simulink model "ensembleSNN_simulink"  (R2019a)
settings: Solver=FixedStepAuto  StartTime=0.0  StopTime=12  FixedStep=0.001  RelTol=1e-3
libraries: simulink x2, dspsigops x1
(part 3 of 3)

== system ensembleSNN_simulink/izhiekvichNeuron6/u' switch ==
  In1 : Inport
  In2 : Inport  Port=2
  In3 : Inport  Port=3
  Switch Delay - 3 : Delay  DelayLength=3
  Switch4 : Switch  Criteria=u2 > Threshold  Threshold=30
  Out1 : Outport  VectorParamsAs1DForOutWhenUnconnected=on
  wires:
  In2/1 -> Switch4/2
  Switch4/1 -> Switch Delay - 3/1
  In1/1 -> Switch4/1
  Switch Delay - 3/1 -> Out1/1
  In3/1 -> Switch4/3

== system ensembleSNN_simulink/izhiekvichNeuron6/v + [0.04v2 +5v - u + j +140 ==
  In1 : Inport
  J : Inport  Port=2
  Add : Sum
  Add Delay - 2 : Delay
  Out1 : Outport  VectorParamsAs1DForOutWhenUnconnected=on
  wires:
  Add Delay - 2/1 -> Out1/1
  Add/1 -> Add Delay - 2/1
  In1/1 -> Add/1
  J/1 -> Add/2

== system ensembleSNN_simulink/izhiekvichNeuron6/v' switch ==
  In1 : Inport
  In2 : Inport  Port=2
  In3 : Inport  Port=3
  Switch Delay - 3 : Delay  DelayLength=3
  Switch4 : Switch  Criteria=u2 > Threshold  Threshold=30
  J : Outport  VectorParamsAs1DForOutWhenUnconnected=on
  wires:
  In2/1 -> Switch4/2
  Switch4/1 -> Switch Delay - 3/1
  In1/1 -> Switch4/1
  Switch Delay - 3/1 -> J/1
  In3/1 -> Switch4/3

== system ensembleSNN_simulink/izhiekvichNeuron6/v^2 ==
  J : Inport
  In2 : Inport  Port=2
  Mult Delay - 2 : Delay  DelayLength=1
  Product1 : Product
  Out1 : Outport  VectorParamsAs1DForOutWhenUnconnected=on
  wires:
  Product1/1 -> Mult Delay - 2/1
  In2/1 -> Product1/2
  J/1 -> Product1/1
  Mult Delay - 2/1 -> Out1/1

== system ensembleSNN_simulink/izhiekvichNeuron7/0.04v2 +5v - u ==
  In1 : Inport
  In2 : Inport  Port=2
  Subtract : Sum  Inputs=+-
  Subtract Delay - 1 : Delay  DelayLength=1
  Out1 : Outport  VectorParamsAs1DForOutWhenUnconnected=on
  wires:
  In1/1 -> Subtract/1
  Subtract/1 -> Subtract Delay - 1/1
  Subtract Delay - 1/1 -> Out1/1
  In2/1 -> Subtract/2

== system ensembleSNN_simulink/izhiekvichNeuron7/0.04v2 +5v - u + j +140 ==
  In1 : Inport
  J : Inport  Port=2
  Add : Sum
  Add Delay - 2 : Delay
  Out1 : Outport  VectorParamsAs1DForOutWhenUnconnected=on
  wires:
  Add Delay - 2/1 -> Out1/1
  Add/1 -> Add Delay - 2/1
  In1/1 -> Add/1
  J/1 -> Add/2

== system ensembleSNN_simulink/izhiekvichNeuron7/0.04v^2 ==
  In1 : Inport
  In2 : Inport  Port=2
  Mult Delay - 1 : Delay  DelayLength=1
  Product1 : Product
  Out1 : Outport  VectorParamsAs1DForOutWhenUnconnected=on
  wires:
  Product1/1 -> Mult Delay - 1/1
  Mult Delay - 1/1 -> Out1/1
  In2/1 -> Product1/2
  In1/1 -> Product1/1

== system ensembleSNN_simulink/izhiekvichNeuron7/0.04v^2 +5v ==
  In1 : Inport
  In2 : Inport  Port=2
  Add : Sum
  Add Delay - 2 : Delay
  Out1 : Outport  VectorParamsAs1DForOutWhenUnconnected=on
  wires:
  Add Delay - 2/1 -> Out1/1
  Add/1 -> Add Delay - 2/1
  In1/1 -> Add/1
  In2/1 -> Add/2

== system ensembleSNN_simulink/izhiekvichNeuron7/5v ==
  J : Inport
  In2 : Inport  Port=2
  Mult Delay - 1 : Delay  DelayLength=1
  Product1 : Product
  Out1 : Outport  VectorParamsAs1DForOutWhenUnconnected=on
  wires:
  Product1/1 -> Mult Delay - 1/1
  Mult Delay - 1/1 -> Out1/1
  In2/1 -> Product1/2
  J/1 -> Product1/1

== system ensembleSNN_simulink/izhiekvichNeuron7/a(bv-u) ==
  In1 : Inport
  In2 : Inport  Port=2
  Mult Delay - 1 : Delay  DelayLength=1
  Product1 : Product
  Out1 : Outport  VectorParamsAs1DForOutWhenUnconnected=on
  wires:
  Product1/1 -> Mult Delay - 1/1
  Mult Delay - 1/1 -> Out1/1
  In2/1 -> Product1/2
  In1/1 -> Product1/1

== system ensembleSNN_simulink/izhiekvichNeuron7/bv ==
  In1 : Inport
  J : Inport  Port=2
  Mult Delay - 1 : Delay  DelayLength=1
  Product1 : Product
  Out1 : Outport  VectorParamsAs1DForOutWhenUnconnected=on
  wires:
  Product1/1 -> Mult Delay - 1/1
  Mult Delay - 1/1 -> Out1/1
  J/1 -> Product1/2
  In1/1 -> Product1/1

== system ensembleSNN_simulink/izhiekvichNeuron7/bv - u ==
  In1 : Inport
  In2 : Inport  Port=2
  Subtract : Sum  Inputs=+-
  Subtract Delay - 1 : Delay  DelayLength=1
  Out1 : Outport  VectorParamsAs1DForOutWhenUnconnected=on
  wires:
  In1/1 -> Subtract/1
  Subtract/1 -> Subtract Delay - 1/1
  Subtract Delay - 1/1 -> Out1/1
  In2/1 -> Subtract/2

== system ensembleSNN_simulink/izhiekvichNeuron7/j + 140 ==
  In1 : Inport
  J : Inport  Port=2
  Add : Sum
  Add Delay - 2 : Delay
  Out1 : Outport  VectorParamsAs1DForOutWhenUnconnected=on
  wires:
  Add Delay - 2/1 -> Out1/1
  Add/1 -> Add Delay - 2/1
  In1/1 -> Add/1
  J/1 -> Add/2

== system ensembleSNN_simulink/izhiekvichNeuron7/u + a(bv-u) ==
  In1 : Inport
  In2 : Inport  Port=2
  Add : Sum
  Add Delay - 2 : Delay
  Out1 : Outport  VectorParamsAs1DForOutWhenUnconnected=on
  wires:
  Add Delay - 2/1 -> Out1/1
  Add/1 -> Add Delay - 2/1
  In1/1 -> Add/1
  In2/1 -> Add/2

== system ensembleSNN_simulink/izhiekvichNeuron7/u' + d ==
  In1 : Inport
  In2 : Inport  Port=2
  Add : Sum
  Add Delay - 2 : Delay
  Out1 : Outport  VectorParamsAs1DForOutWhenUnconnected=on
  wires:
  Add Delay - 2/1 -> Out1/1
  Add/1 -> Add Delay - 2/1
  In1/1 -> Add/1
  In2/1 -> Add/2

== system ensembleSNN_simulink/izhiekvichNeuron7/u' switch ==
  In1 : Inport
  In2 : Inport  Port=2
  In3 : Inport  Port=3
  Switch Delay - 3 : Delay  DelayLength=3
  Switch4 : Switch  Criteria=u2 > Threshold  Threshold=30
  Out1 : Outport  VectorParamsAs1DForOutWhenUnconnected=on
  wires:
  In2/1 -> Switch4/2
  Switch4/1 -> Switch Delay - 3/1
  In1/1 -> Switch4/1
  Switch Delay - 3/1 -> Out1/1
  In3/1 -> Switch4/3

== system ensembleSNN_simulink/izhiekvichNeuron7/v + [0.04v2 +5v - u + j +140 ==
  In1 : Inport
  J : Inport  Port=2
  Add : Sum
  Add Delay - 2 : Delay
  Out1 : Outport  VectorParamsAs1DForOutWhenUnconnected=on
  wires:
  Add Delay - 2/1 -> Out1/1
  Add/1 -> Add Delay - 2/1
  In1/1 -> Add/1
  J/1 -> Add/2

== system ensembleSNN_simulink/izhiekvichNeuron7/v' switch ==
  In1 : Inport
  In2 : Inport  Port=2
  In3 : Inport  Port=3
  Switch Delay - 3 : Delay  DelayLength=3
  Switch4 : Switch  Criteria=u2 > Threshold  Threshold=30
  J : Outport  VectorParamsAs1DForOutWhenUnconnected=on
  wires:
  In2/1 -> Switch4/2
  Switch4/1 -> Switch Delay - 3/1
  In1/1 -> Switch4/1
  Switch Delay - 3/1 -> J/1
  In3/1 -> Switch4/3

== system ensembleSNN_simulink/izhiekvichNeuron7/v^2 ==
  J : Inport
  In2 : Inport  Port=2
  Mult Delay - 2 : Delay  DelayLength=1
  Product1 : Product
  Out1 : Outport  VectorParamsAs1DForOutWhenUnconnected=on
  wires:
  Product1/1 -> Mult Delay - 2/1
  In2/1 -> Product1/2
  J/1 -> Product1/1
  Mult Delay - 2/1 -> Out1/1

== system ensembleSNN_simulink/izhiekvichNeuron8/0.04v2 +5v - u ==
  In1 : Inport
  In2 : Inport  Port=2
  Subtract : Sum  Inputs=+-
  Subtract Delay - 1 : Delay  DelayLength=1
  Out1 : Outport  VectorParamsAs1DForOutWhenUnconnected=on
  wires:
  In1/1 -> Subtract/1
  Subtract/1 -> Subtract Delay - 1/1
  Subtract Delay - 1/1 -> Out1/1
  In2/1 -> Subtract/2

== system ensembleSNN_simulink/izhiekvichNeuron8/0.04v2 +5v - u + j +140 ==
  In1 : Inport
  J : Inport  Port=2
  Add : Sum
  Add Delay - 2 : Delay
  Out1 : Outport  VectorParamsAs1DForOutWhenUnconnected=on
  wires:
  Add Delay - 2/1 -> Out1/1
  Add/1 -> Add Delay - 2/1
  In1/1 -> Add/1
  J/1 -> Add/2

== system ensembleSNN_simulink/izhiekvichNeuron8/0.04v^2 ==
  In1 : Inport
  In2 : Inport  Port=2
  Mult Delay - 1 : Delay  DelayLength=1
  Product1 : Product
  Out1 : Outport  VectorParamsAs1DForOutWhenUnconnected=on
  wires:
  Product1/1 -> Mult Delay - 1/1
  Mult Delay - 1/1 -> Out1/1
  In2/1 -> Product1/2
  In1/1 -> Product1/1

== system ensembleSNN_simulink/izhiekvichNeuron8/0.04v^2 +5v ==
  In1 : Inport
  In2 : Inport  Port=2
  Add : Sum
  Add Delay - 2 : Delay
  Out1 : Outport  VectorParamsAs1DForOutWhenUnconnected=on
  wires:
  Add Delay - 2/1 -> Out1/1
  Add/1 -> Add Delay - 2/1
  In1/1 -> Add/1
  In2/1 -> Add/2

== system ensembleSNN_simulink/izhiekvichNeuron8/5v ==
  J : Inport
  In2 : Inport  Port=2
  Mult Delay - 1 : Delay  DelayLength=1
  Product1 : Product
  Out1 : Outport  VectorParamsAs1DForOutWhenUnconnected=on
  wires:
  Product1/1 -> Mult Delay - 1/1
  Mult Delay - 1/1 -> Out1/1
  In2/1 -> Product1/2
  J/1 -> Product1/1

== system ensembleSNN_simulink/izhiekvichNeuron8/a(bv-u) ==
  In1 : Inport
  In2 : Inport  Port=2
  Mult Delay - 1 : Delay  DelayLength=1
  Product1 : Product
  Out1 : Outport  VectorParamsAs1DForOutWhenUnconnected=on
  wires:
  Product1/1 -> Mult Delay - 1/1
  Mult Delay - 1/1 -> Out1/1
  In2/1 -> Product1/2
  In1/1 -> Product1/1

== system ensembleSNN_simulink/izhiekvichNeuron8/bv ==
  In1 : Inport
  J : Inport  Port=2
  Mult Delay - 1 : Delay  DelayLength=1
  Product1 : Product
  Out1 : Outport  VectorParamsAs1DForOutWhenUnconnected=on
  wires:
  Product1/1 -> Mult Delay - 1/1
  Mult Delay - 1/1 -> Out1/1
  J/1 -> Product1/2
  In1/1 -> Product1/1

== system ensembleSNN_simulink/izhiekvichNeuron8/bv - u ==
  In1 : Inport
  In2 : Inport  Port=2
  Subtract : Sum  Inputs=+-
  Subtract Delay - 1 : Delay  DelayLength=1
  Out1 : Outport  VectorParamsAs1DForOutWhenUnconnected=on
  wires:
  In1/1 -> Subtract/1
  Subtract/1 -> Subtract Delay - 1/1
  Subtract Delay - 1/1 -> Out1/1
  In2/1 -> Subtract/2

== system ensembleSNN_simulink/izhiekvichNeuron8/j + 140 ==
  In1 : Inport
  J : Inport  Port=2
  Add : Sum
  Add Delay - 2 : Delay
  Out1 : Outport  VectorParamsAs1DForOutWhenUnconnected=on
  wires:
  Add Delay - 2/1 -> Out1/1
  Add/1 -> Add Delay - 2/1
  In1/1 -> Add/1
  J/1 -> Add/2

== system ensembleSNN_simulink/izhiekvichNeuron8/u + a(bv-u) ==
  In1 : Inport
  In2 : Inport  Port=2
  Add : Sum
  Add Delay - 2 : Delay
  Out1 : Outport  VectorParamsAs1DForOutWhenUnconnected=on
  wires:
  Add Delay - 2/1 -> Out1/1
  Add/1 -> Add Delay - 2/1
  In1/1 -> Add/1
  In2/1 -> Add/2

== system ensembleSNN_simulink/izhiekvichNeuron8/u' + d ==
  In1 : Inport
  In2 : Inport  Port=2
  Add : Sum
  Add Delay - 2 : Delay
  Out1 : Outport  VectorParamsAs1DForOutWhenUnconnected=on
  wires:
  Add Delay - 2/1 -> Out1/1
  Add/1 -> Add Delay - 2/1
  In1/1 -> Add/1
  In2/1 -> Add/2

== system ensembleSNN_simulink/izhiekvichNeuron8/u' switch ==
  In1 : Inport
  In2 : Inport  Port=2
  In3 : Inport  Port=3
  Switch Delay - 3 : Delay  DelayLength=3
  Switch4 : Switch  Criteria=u2 > Threshold  Threshold=30
  Out1 : Outport  VectorParamsAs1DForOutWhenUnconnected=on
  wires:
  In2/1 -> Switch4/2
  Switch4/1 -> Switch Delay - 3/1
  In1/1 -> Switch4/1
  Switch Delay - 3/1 -> Out1/1
  In3/1 -> Switch4/3

== system ensembleSNN_simulink/izhiekvichNeuron8/v + [0.04v2 +5v - u + j +140 ==
  In1 : Inport
  J : Inport  Port=2
  Add : Sum
  Add Delay - 2 : Delay
  Out1 : Outport  VectorParamsAs1DForOutWhenUnconnected=on
  wires:
  Add Delay - 2/1 -> Out1/1
  Add/1 -> Add Delay - 2/1
  In1/1 -> Add/1
  J/1 -> Add/2

== system ensembleSNN_simulink/izhiekvichNeuron8/v' switch ==
  In1 : Inport
  In2 : Inport  Port=2
  In3 : Inport  Port=3
  Switch Delay - 3 : Delay  DelayLength=3
  Switch4 : Switch  Criteria=u2 > Threshold  Threshold=30
  J : Outport  VectorParamsAs1DForOutWhenUnconnected=on
  wires:
  In2/1 -> Switch4/2
  Switch4/1 -> Switch Delay - 3/1
  In1/1 -> Switch4/1
  Switch Delay - 3/1 -> J/1
  In3/1 -> Switch4/3

== system ensembleSNN_simulink/izhiekvichNeuron8/v^2 ==
  J : Inport
  In2 : Inport  Port=2
  Mult Delay - 2 : Delay  DelayLength=1
  Product1 : Product
  Out1 : Outport  VectorParamsAs1DForOutWhenUnconnected=on
  wires:
  Product1/1 -> Mult Delay - 2/1
  In2/1 -> Product1/2
  J/1 -> Product1/1
  Mult Delay - 2/1 -> Out1/1

== system ensembleSNN_simulink/izhiekvichNeuron9/0.04v2 +5v - u ==
  In1 : Inport
  In2 : Inport  Port=2
  Subtract : Sum  Inputs=+-
  Subtract Delay - 1 : Delay  DelayLength=1
  Out1 : Outport  VectorParamsAs1DForOutWhenUnconnected=on
  wires:
  In1/1 -> Subtract/1
  Subtract/1 -> Subtract Delay - 1/1
  Subtract Delay - 1/1 -> Out1/1
  In2/1 -> Subtract/2

== system ensembleSNN_simulink/izhiekvichNeuron9/0.04v2 +5v - u + j +140 ==
  In1 : Inport
  J : Inport  Port=2
  Add : Sum
  Add Delay - 2 : Delay
  Out1 : Outport  VectorParamsAs1DForOutWhenUnconnected=on
  wires:
  Add Delay - 2/1 -> Out1/1
  Add/1 -> Add Delay - 2/1
  In1/1 -> Add/1
  J/1 -> Add/2

== system ensembleSNN_simulink/izhiekvichNeuron9/0.04v^2 ==
  In1 : Inport
  In2 : Inport  Port=2
  Mult Delay - 1 : Delay  DelayLength=1
  Product1 : Product
  Out1 : Outport  VectorParamsAs1DForOutWhenUnconnected=on
  wires:
  Product1/1 -> Mult Delay - 1/1
  Mult Delay - 1/1 -> Out1/1
  In2/1 -> Product1/2
  In1/1 -> Product1/1

== system ensembleSNN_simulink/izhiekvichNeuron9/0.04v^2 +5v ==
  In1 : Inport
  In2 : Inport  Port=2
  Add : Sum
  Add Delay - 2 : Delay
  Out1 : Outport  VectorParamsAs1DForOutWhenUnconnected=on
  wires:
  Add Delay - 2/1 -> Out1/1
  Add/1 -> Add Delay - 2/1
  In1/1 -> Add/1
  In2/1 -> Add/2

== system ensembleSNN_simulink/izhiekvichNeuron9/5v ==
  J : Inport
  In2 : Inport  Port=2
  Mult Delay - 1 : Delay  DelayLength=1
  Product1 : Product
  Out1 : Outport  VectorParamsAs1DForOutWhenUnconnected=on
  wires:
  Product1/1 -> Mult Delay - 1/1
  Mult Delay - 1/1 -> Out1/1
  In2/1 -> Product1/2
  J/1 -> Product1/1

== system ensembleSNN_simulink/izhiekvichNeuron9/a(bv-u) ==
  In1 : Inport
  In2 : Inport  Port=2
  Mult Delay - 1 : Delay  DelayLength=1
  Product1 : Product
  Out1 : Outport  VectorParamsAs1DForOutWhenUnconnected=on
  wires:
  Product1/1 -> Mult Delay - 1/1
  Mult Delay - 1/1 -> Out1/1
  In2/1 -> Product1/2
  In1/1 -> Product1/1

== system ensembleSNN_simulink/izhiekvichNeuron9/bv ==
  In1 : Inport
  J : Inport  Port=2
  Mult Delay - 1 : Delay  DelayLength=1
  Product1 : Product
  Out1 : Outport  VectorParamsAs1DForOutWhenUnconnected=on
  wires:
  Product1/1 -> Mult Delay - 1/1
  Mult Delay - 1/1 -> Out1/1
  J/1 -> Product1/2
  In1/1 -> Product1/1

== system ensembleSNN_simulink/izhiekvichNeuron9/bv - u ==
  In1 : Inport
  In2 : Inport  Port=2
  Subtract : Sum  Inputs=+-
  Subtract Delay - 1 : Delay  DelayLength=1
  Out1 : Outport  VectorParamsAs1DForOutWhenUnconnected=on
  wires:
  In1/1 -> Subtract/1
  Subtract/1 -> Subtract Delay - 1/1
  Subtract Delay - 1/1 -> Out1/1
  In2/1 -> Subtract/2

== system ensembleSNN_simulink/izhiekvichNeuron9/j + 140 ==
  In1 : Inport
  J : Inport  Port=2
  Add : Sum
  Add Delay - 2 : Delay
  Out1 : Outport  VectorParamsAs1DForOutWhenUnconnected=on
  wires:
  Add Delay - 2/1 -> Out1/1
  Add/1 -> Add Delay - 2/1
  In1/1 -> Add/1
  J/1 -> Add/2

== system ensembleSNN_simulink/izhiekvichNeuron9/u + a(bv-u) ==
  In1 : Inport
  In2 : Inport  Port=2
  Add : Sum
  Add Delay - 2 : Delay
  Out1 : Outport  VectorParamsAs1DForOutWhenUnconnected=on
  wires:
  Add Delay - 2/1 -> Out1/1
  Add/1 -> Add Delay - 2/1
  In1/1 -> Add/1
  In2/1 -> Add/2

== system ensembleSNN_simulink/izhiekvichNeuron9/u' + d ==
  In1 : Inport
  In2 : Inport  Port=2
  Add : Sum
  Add Delay - 2 : Delay
  Out1 : Outport  VectorParamsAs1DForOutWhenUnconnected=on
  wires:
  Add Delay - 2/1 -> Out1/1
  Add/1 -> Add Delay - 2/1
  In1/1 -> Add/1
  In2/1 -> Add/2

== system ensembleSNN_simulink/izhiekvichNeuron9/u' switch ==
  In1 : Inport
  In2 : Inport  Port=2
  In3 : Inport  Port=3
  Switch Delay - 3 : Delay  DelayLength=3
  Switch4 : Switch  Criteria=u2 > Threshold  Threshold=30
  Out1 : Outport  VectorParamsAs1DForOutWhenUnconnected=on
  wires:
  In2/1 -> Switch4/2
  Switch4/1 -> Switch Delay - 3/1
  In1/1 -> Switch4/1
  Switch Delay - 3/1 -> Out1/1
  In3/1 -> Switch4/3

== system ensembleSNN_simulink/izhiekvichNeuron9/v + [0.04v2 +5v - u + j +140 ==
  In1 : Inport
  J : Inport  Port=2
  Add : Sum
  Add Delay - 2 : Delay
  Out1 : Outport  VectorParamsAs1DForOutWhenUnconnected=on
  wires:
  Add Delay - 2/1 -> Out1/1
  Add/1 -> Add Delay - 2/1
  In1/1 -> Add/1
  J/1 -> Add/2

== system ensembleSNN_simulink/izhiekvichNeuron9/v' switch ==
  In1 : Inport
  In2 : Inport  Port=2
  In3 : Inport  Port=3
  Switch Delay - 3 : Delay  DelayLength=3
  Switch4 : Switch  Criteria=u2 > Threshold  Threshold=30
  J : Outport  VectorParamsAs1DForOutWhenUnconnected=on
  wires:
  In2/1 -> Switch4/2
  Switch4/1 -> Switch Delay - 3/1
  In1/1 -> Switch4/1
  Switch Delay - 3/1 -> J/1
  In3/1 -> Switch4/3

== system ensembleSNN_simulink/izhiekvichNeuron9/v^2 ==
  J : Inport
  In2 : Inport  Port=2
  Mult Delay - 2 : Delay  DelayLength=1
  Product1 : Product
  Out1 : Outport  VectorParamsAs1DForOutWhenUnconnected=on
  wires:
  Product1/1 -> Mult Delay - 2/1
  In2/1 -> Product1/2
  J/1 -> Product1/1
  Mult Delay - 2/1 -> Out1/1
